simulink model "PMSM_id_iq_Regelung"  (R2014b)
settings: Solver=ode4  StartTime=0.0  StopTime=5  FixedStep=5e-6  RelTol=1e-3
undefined symbols (not defined in the file): J, Ld, Lq, p, Psi_pm, R1
settings Model: Creator=benjamin  LastModifiedBy=Benji

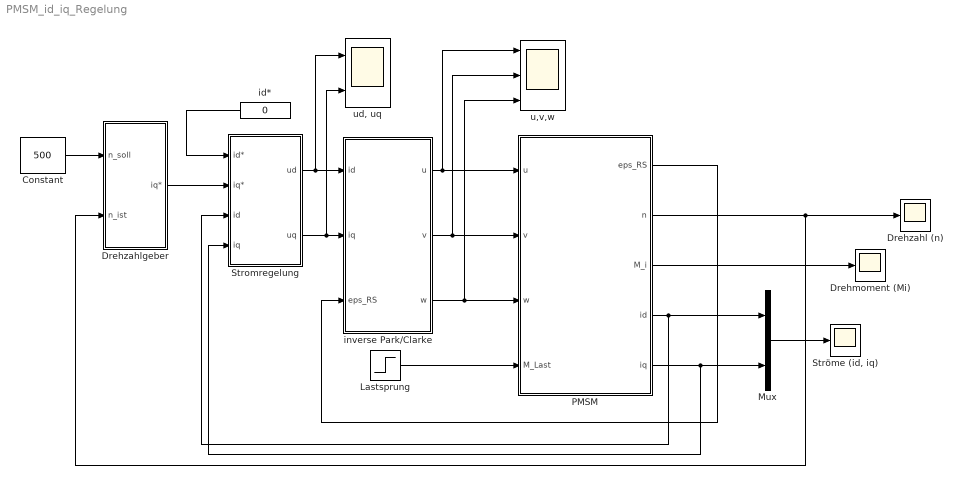
== system PMSM_id_iq_Regelung ==
  Constant : Constant  Value=500
  Drehmoment (Mi) : Scope
      settings: SaveName=ScopeData2
  Drehzahl (n) : Scope
      settings: TimeRange=5  YMin=0  YMax=600  SaveName=ScopeData3
  Drehzahlgeber : Subsystem
  Lastsprung : Step  Time=3  After=60  SampleTime=0
  Mux : Mux  Inputs=2
  PMSM : Subsystem
  Stromregelung : Subsystem
  "Ströme (id, iq)" : Scope
      settings: SaveName=ScopeData4
  id* : Constant  Value=0
  inverse Park/Clarke : Subsystem
  u,v,w : Scope  NumInputPorts=3
      settings: YMin=0~-100~-5  YMax=900~100~5  SaveName=ScopeData5
  "ud, uq" : Scope  NumInputPorts=2
      settings: YMin=0~-100  YMax=900~100
  wires:
  id*/1 -> Stromregelung/1(id*)
  Drehzahlgeber/1(iq*) -> Stromregelung/2(iq*)
  Constant/1 -> Drehzahlgeber/1(n_soll)
  PMSM/4(id) -> Stromregelung/3(id), Mux/1
  PMSM/5(iq) -> Stromregelung/4(iq), Mux/2
  PMSM/2(n) -> Drehzahl (n)/1, Drehzahlgeber/2(n_ist)
  inverse Park/Clarke/1(u) -> u,v,w/1, PMSM/1("u ")
  inverse Park/Clarke/2(v) -> u,v,w/2, PMSM/2(v)
  inverse Park/Clarke/3(w) -> u,v,w/3, PMSM/3(w)
  Stromregelung/1(ud) -> "ud, uq"/1, inverse Park/Clarke/1(id)
  Stromregelung/2(uq) -> "ud, uq"/2, inverse Park/Clarke/2(iq)
  PMSM/1(eps_RS) -> inverse Park/Clarke/3(eps_RS)
  Lastsprung/1 -> PMSM/4(M_Last)
  PMSM/3(M_i) -> Drehmoment (Mi)/1
  Mux/1 -> "Ströme (id, iq)"/1

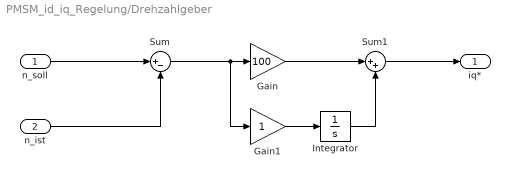
== system PMSM_id_iq_Regelung/Drehzahlgeber ==
  n_soll : Inport
  n_ist : Inport  Port=2
  Gain : Gain  Gain=100
  Gain1 : Gain
  Integrator : Integrator
  Sum : Sum  Inputs=|+-
  Sum1 : Sum  Inputs=|++
  iq* : Outport
  wires:
  n_soll/1 -> Sum/1
  n_ist/1 -> Sum/2
  Sum/1 -> Gain1/1, Gain/1
  Gain/1 -> Sum1/1
  Gain1/1 -> Integrator/1
  Integrator/1 -> Sum1/2
  Sum1/1 -> iq*/1

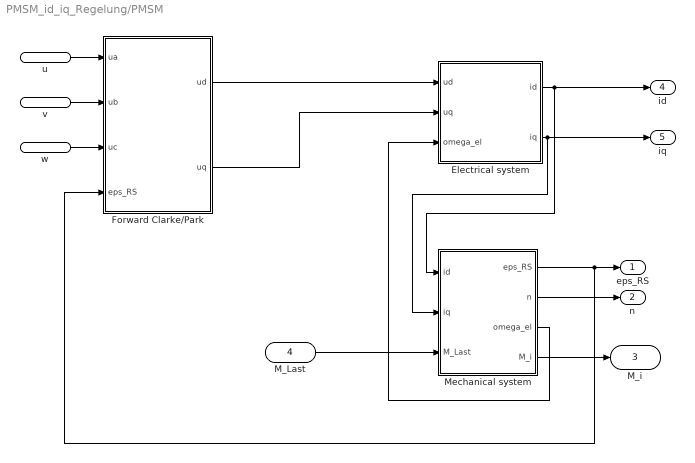
== system PMSM_id_iq_Regelung/PMSM ==
  "u " : Inport
  v : Inport  Port=2
  w : Inport  Port=3
  M_Last : Inport  Port=4
  Electrical system : Subsystem
  Forward Clarke/Park : Subsystem
  Mechanical system : Subsystem
  eps_RS : Outport
  n : Outport  Port=2
  M_i : Outport  Port=3
  id : Outport  Port=4
  iq : Outport  Port=5
  wires:
  Electrical system/1(id) -> id/1, Mechanical system/1(id)
  Electrical system/2(iq) -> iq/1, Mechanical system/2(iq)
  Mechanical system/3(omega_el) -> Electrical system/3(omega_el)
  Mechanical system/1(eps_RS) -> Forward Clarke/Park/4(eps_RS), eps_RS/1
  Mechanical system/2(n) -> n/1
  Mechanical system/4(M_i) -> M_i/1
  M_Last/1 -> Mechanical system/3(M_Last)
  "u "/1 -> Forward Clarke/Park/1(ua)
  v/1 -> Forward Clarke/Park/2(ub)
  w/1 -> Forward Clarke/Park/3(uc)
  Forward Clarke/Park/1(ud) -> Electrical system/1(ud)
  Forward Clarke/Park/2(uq) -> Electrical system/2(uq)

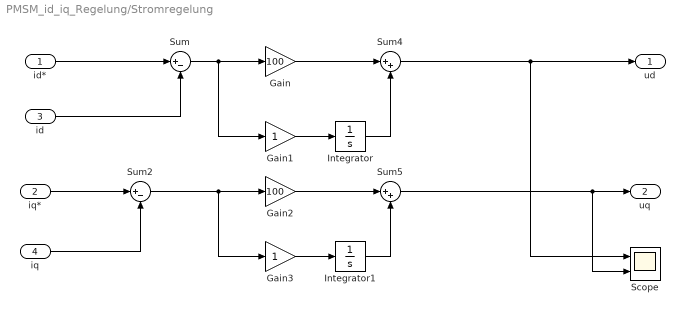
== system PMSM_id_iq_Regelung/Stromregelung ==
  id* : Inport
  iq* : Inport  Port=2
  id : Inport  Port=3
  iq : Inport  Port=4
  Gain : Gain  Gain=100
  Gain1 : Gain
  Gain2 : Gain  Gain=100
  Gain3 : Gain
  Integrator : Integrator
  Integrator1 : Integrator
  Scope : Scope  NumInputPorts=2
      settings: TimeRange=5  YMin=-1.3~-5  YMax=0~5
  Sum : Sum  Inputs=|+-
  Sum2 : Sum  Inputs=|+-
  Sum4 : Sum  Inputs=|++
  Sum5 : Sum  Inputs=|++
  ud : Outport
  uq : Outport  Port=2
  wires:
  iq*/1 -> Sum2/1
  id*/1 -> Sum/1
  id/1 -> Sum/2
  iq/1 -> Sum2/2
  Sum/1 -> Gain1/1, Gain/1
  Gain/1 -> Sum4/1
  Gain1/1 -> Integrator/1
  Integrator/1 -> Sum4/2
  Sum2/1 -> Gain3/1, Gain2/1
  Gain2/1 -> Sum5/1
  Gain3/1 -> Integrator1/1
  Integrator1/1 -> Sum5/2
  Sum5/1 -> Scope/2, uq/1
  Sum4/1 -> ud/1, Scope/1

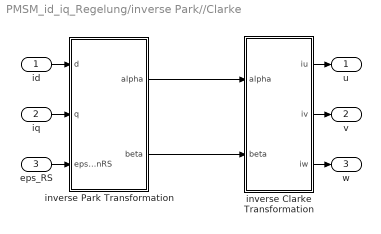
== system PMSM_id_iq_Regelung/inverse Park//Clarke ==
  id : Inport
  iq : Inport  Port=2
  eps_RS : Inport  Port=3
  inverse Clarke Transformation : Subsystem
  inverse Park Transformation : Subsystem
  u : Outport
  v : Outport  Port=2
  w : Outport  Port=3
  wires:
  inverse Park Transformation/1(alpha) -> inverse Clarke Transformation/1(alpha)
  inverse Park Transformation/2(beta) -> inverse Clarke Transformation/2(beta)
  inverse Clarke Transformation/1(iu) -> u/1
  id/1 -> inverse Park Transformation/1(d)
  iq/1 -> inverse Park Transformation/2(q)
  eps_RS/1 -> inverse Park Transformation/3(epsilonRS)
  inverse Clarke Transformation/2(iv) -> v/1
  inverse Clarke Transformation/3(iw) -> w/1

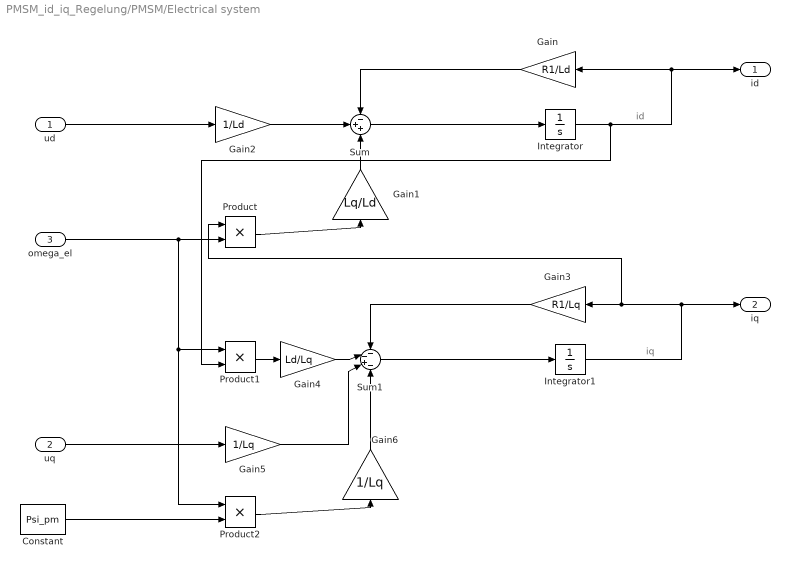
== system PMSM_id_iq_Regelung/PMSM/Electrical system ==
  note: id
  note: iq
  ud : Inport
  uq : Inport  Port=2
  omega_el : Inport  Port=3
  Constant : Constant  Value=Psi_pm
  Gain : Gain  Gain=R1/Ld
  Gain1 : Gain  Gain=Lq/Ld
  Gain2 : Gain  Gain=1/Ld
  Gain3 : Gain  Gain=R1/Lq
  Gain4 : Gain  Gain=Ld/Lq
  Gain5 : Gain  Gain=1/Lq
  Gain6 : Gain  Gain=1/Lq
  Integrator : Integrator
  Integrator1 : Integrator
  Product : Product
  Product1 : Product
  Product2 : Product
  Sum : Sum  Inputs=-++
  Sum1 : Sum  Inputs=--+-
  id : Outport
  iq : Outport  Port=2
  wires:
  Sum/1 -> Integrator/1
  Integrator/1 -> Product1/2, Gain/1, id/1
  Gain/1 -> Sum/1
  omega_el/1 -> Product2/1, Product1/1, Product/2
  Gain1/1 -> Sum/3
  Product/1 -> Gain1/1
  ud/1 -> Gain2/1
  Gain2/1 -> Sum/2
  Sum1/1 -> Integrator1/1
  Integrator1/1 -> iq/1, Product/1, Gain3/1
  Gain3/1 -> Sum1/1
  Gain5/1 -> Sum1/3
  Product1/1 -> Gain4/1
  Gain4/1 -> Sum1/2
  uq/1 -> Gain5/1
  Constant/1 -> Product2/2
  Gain6/1 -> Sum1/4
  Product2/1 -> Gain6/1

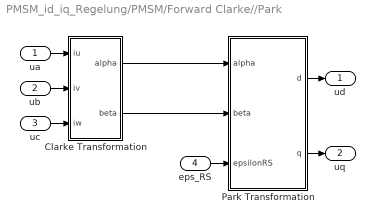
== system PMSM_id_iq_Regelung/PMSM/Forward Clarke//Park ==
  ua : Inport
  ub : Inport  Port=2
  uc : Inport  Port=3
  eps_RS : Inport  Port=4
  Clarke Transformation : Subsystem
  Park Transformation : Subsystem
  ud : Outport
  uq : Outport  Port=2
  wires:
  ua/1 -> Clarke Transformation/1(iu)
  Clarke Transformation/1(alpha) -> Park Transformation/1(alpha)
  Clarke Transformation/2(beta) -> Park Transformation/2(beta)
  eps_RS/1 -> Park Transformation/3(epsilonRS)
  Park Transformation/1(d) -> ud/1
  uc/1 -> Clarke Transformation/3(iw)
  Park Transformation/2(q) -> uq/1
  ub/1 -> Clarke Transformation/2(iv)

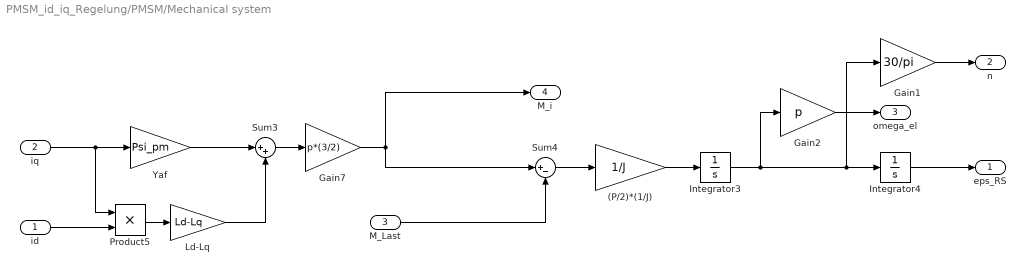
== system PMSM_id_iq_Regelung/PMSM/Mechanical system ==
  id : Inport
  iq : Inport  Port=2
  M_Last : Inport  Port=3
  (P/2)*(1/J) : Gain  Gain=1/J
  Gain1 : Gain  Gain=30/pi
  Gain2 : Gain  Gain=p
  Gain7 : Gain  Gain=p*(3/2)
  Integrator3 : Integrator
  Integrator4 : Integrator
  Ld-Lq : Gain  Gain=Ld-Lq
  Product5 : Product  RndMeth=Zero
  Sum3 : Sum  Inputs=|++
  Sum4 : Sum  Inputs=|+-
  Yaf : Gain  Gain=Psi_pm
  eps_RS : Outport
  n : Outport  Port=2
  omega_el : Outport  Port=3
  M_i : Outport  Port=4
  wires:
  Yaf/1 -> Sum3/1
  Sum3/1 -> Gain7/1
  Ld-Lq/1 -> Sum3/2
  Product5/1 -> Ld-Lq/1
  Sum4/1 -> (P/2)*(1/J)/1
  iq/1 -> Product5/1, Yaf/1
  id/1 -> Product5/2
  Gain7/1 -> Sum4/1, M_i/1
  (P/2)*(1/J)/1 -> Integrator3/1
  Integrator4/1 -> eps_RS/1
  Gain1/1 -> n/1
  Integrator3/1 -> Gain1/1, Integrator4/1, Gain2/1
  M_Last/1 -> Sum4/2
  Gain2/1 -> omega_el/1

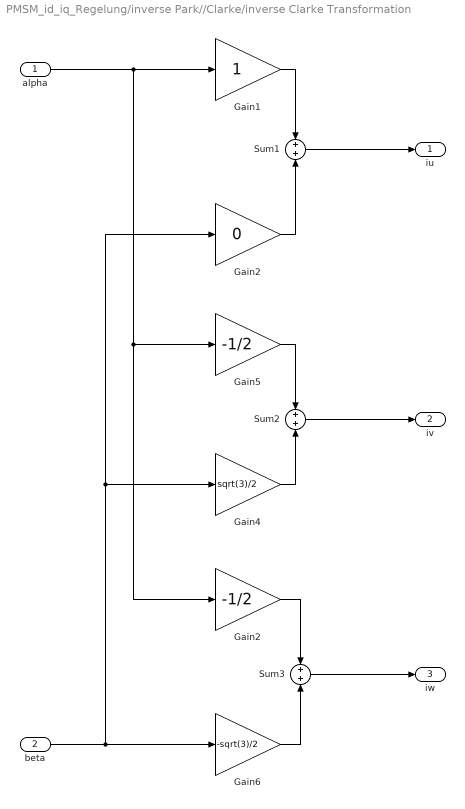
== system PMSM_id_iq_Regelung/inverse Park//Clarke/inverse Clarke Transformation ==
  alpha : Inport
  beta : Inport  Port=2
  Gain1 : Gain
  Gain2 : Gain  Gain=-1/2
  "Gain2 " : Gain  Gain=0
  Gain4 : Gain  Gain=sqrt(3)/2
  Gain5 : Gain  Gain=-1/2
  Gain6 : Gain  Gain=-sqrt(3)/2
  Sum1 : Sum
  Sum2 : Sum
  Sum3 : Sum
  iu : Outport
  iv : Outport  Port=2
  iw : Outport  Port=3
  wires:
  Sum2/1 -> iv/1
  beta/1 -> "Gain2 "/1, Gain4/1, Gain6/1
  Gain4/1 -> Sum2/2
  Sum1/1 -> iu/1
  "Gain2 "/1 -> Sum1/2
  Gain5/1 -> Sum2/1
  Gain1/1 -> Sum1/1
  Gain2/1 -> Sum3/1
  Gain6/1 -> Sum3/2
  alpha/1 -> Gain1/1, Gain2/1, Gain5/1
  Sum3/1 -> iw/1

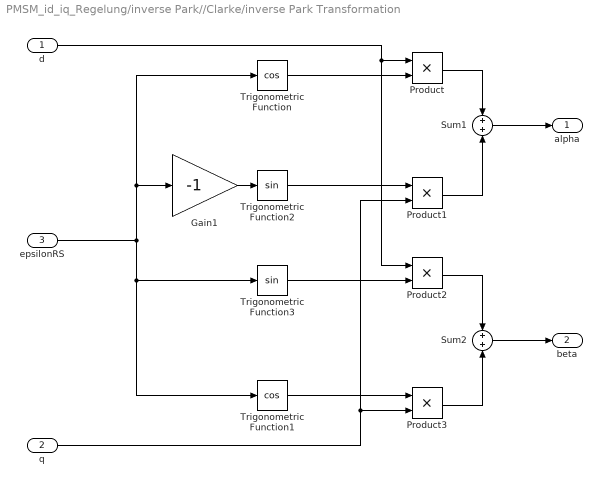
== system PMSM_id_iq_Regelung/inverse Park//Clarke/inverse Park Transformation ==
  d : Inport
  q : Inport  Port=2
  epsilonRS : Inport  Port=3
  Gain1 : Gain  Gain=-1
  Product{,1..3} (4 alike) : Product
  Sum1 : Sum
  Sum2 : Sum
  Trigonometric Function : Trigonometry  Operator=cos
  Trigonometric Function1 : Trigonometry  Operator=cos
  Trigonometric Function2 : Trigonometry
  Trigonometric Function3 : Trigonometry
  alpha : Outport
  beta : Outport  Port=2
  wires:
  Sum2/1 -> beta/1
  Product2/1 -> Sum2/1
  Product1/1 -> Sum1/2
  epsilonRS/1 -> Gain1/1, Trigonometric Function/1, Trigonometric Function3/1, Trigonometric Function1/1
  Trigonometric Function/1 -> Product/2
  d/1 -> Product2/1, Product/1
  Sum1/1 -> alpha/1
  Trigonometric Function1/1 -> Product3/1
  q/1 -> Product3/2, Product1/2
  Product/1 -> Sum1/1
  Trigonometric Function2/1 -> Product1/1
  Trigonometric Function3/1 -> Product2/2
  Product3/1 -> Sum2/2
  Gain1/1 -> Trigonometric Function2/1

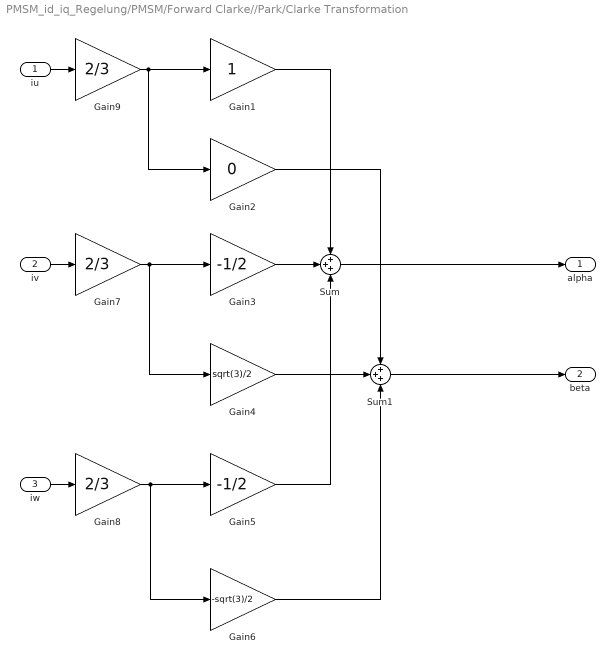
== system PMSM_id_iq_Regelung/PMSM/Forward Clarke//Park/Clarke Transformation ==
  iu : Inport
  iv : Inport  Port=2
  iw : Inport  Port=3
  Gain1 : Gain
  "Gain2 " : Gain  Gain=0
  Gain3 : Gain  Gain=-1/2
  Gain4 : Gain  Gain=sqrt(3)/2
  Gain5 : Gain  Gain=-1/2
  Gain6 : Gain  Gain=-sqrt(3)/2
  Gain7 : Gain  Gain=2/3
  Gain8 : Gain  Gain=2/3
  Gain9 : Gain  Gain=2/3
  Sum : Sum  Inputs=+++
  Sum1 : Sum  Inputs=+++
  alpha : Outport
  beta : Outport  Port=2
  wires:
  "Gain2 "/1 -> Sum1/1
  Gain1/1 -> Sum/1
  Gain4/1 -> Sum1/2
  Gain5/1 -> Sum/3
  iw/1 -> Gain8/1
  Gain3/1 -> Sum/2
  Gain7/1 -> Gain4/1, Gain3/1
  Gain9/1 -> "Gain2 "/1, Gain1/1
  Gain8/1 -> Gain6/1, Gain5/1
  Sum/1 -> alpha/1
  Sum1/1 -> beta/1
  iv/1 -> Gain7/1
  Gain6/1 -> Sum1/3
  iu/1 -> Gain9/1

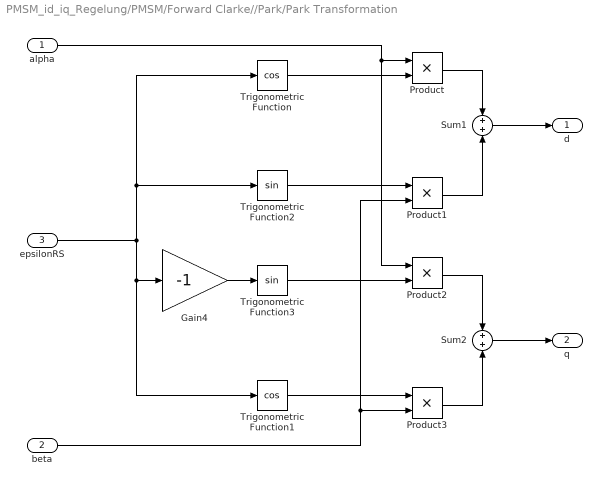
== system PMSM_id_iq_Regelung/PMSM/Forward Clarke//Park/Park Transformation ==
  alpha : Inport
  beta : Inport  Port=2
  epsilonRS : Inport  Port=3
  Gain4 : Gain  Gain=-1
  Product{,1..3} (4 alike) : Product
  Sum1 : Sum
  Sum2 : Sum
  Trigonometric Function : Trigonometry  Operator=cos
  Trigonometric Function1 : Trigonometry  Operator=cos
  Trigonometric Function2 : Trigonometry
  Trigonometric Function3 : Trigonometry
  d : Outport
  q : Outport  Port=2
  wires:
  Sum2/1 -> q/1
  Product2/1 -> Sum2/1
  Product1/1 -> Sum1/2
  epsilonRS/1 -> Trigonometric Function2/1, Trigonometric Function/1, Gain4/1, Trigonometric Function1/1
  Trigonometric Function/1 -> Product/2
  alpha/1 -> Product2/1, Product/1
  Sum1/1 -> d/1
  Trigonometric Function1/1 -> Product3/1
  beta/1 -> Product3/2, Product1/2
  Product/1 -> Sum1/1
  Trigonometric Function2/1 -> Product1/1
  Trigonometric Function3/1 -> Product2/2
  Product3/1 -> Sum2/2
  Gain4/1 -> Trigonometric Function3/1
